simulink model "simulacao1a"  (R2020b)
settings: Solver=VariableStepAuto  StartTime=0.0  StopTime=10  RelTol=1e-3
values from neighbouring files (symbols this model uses):
  b = 0.24    [drone.m]
  B = 0.00029*[1 1 1 1]    [drone.m]
  delta_equilibrium = (Ke(1)*Omega(1) + R(1)*(KQ(1)*Omega(1) + B(1))*Omega(1)/Kt(1))/Vbat    [drone.m]
  J = diag([3.8e-3,3.8e-3,7.1e-3])    [drone.m]
  Jm = 1.4e-5*[1 1 1 1]    [drone.m]
  K = [ Hgain_pd(2) 0             0               0             Hgain_pd(1) 0             0               0 ... (first row only)    [drone.m]
  Ke = 0.0247*[1 1 1 1]    [drone.m]
  KQ = 1.2191e-5*[1 1 1 1]    [drone.m]
  Kt = 0.0247*[1 1 1 1]    [drone.m]
  KT = 3.5897e-5*[1 1 1 1]    [drone.m]
  L = 0.00036*[1 1 1 1]    [drone.m]
  m = 2    [drone.m]
  R = [ cos(target_phi)*cos(target_psi),    cos(target_psi)*sin(target_theta)*sin(target_phi) - sin(target_psi)*cos(target_phi),  cos(target_psi)*sin(target_theta)*cos(target_phi) + sin(target_psi)*sin(target_phi) ... (first row only)    [drone.m]
  Vbat = 15    [drone.m]
libraries: dspmtrx3 x19, vrlib x2
settings Model: Creator=55159  LastModifiedBy=55159
settings DebuggingCC: UnderSpecifiedDimensionMsg=warning

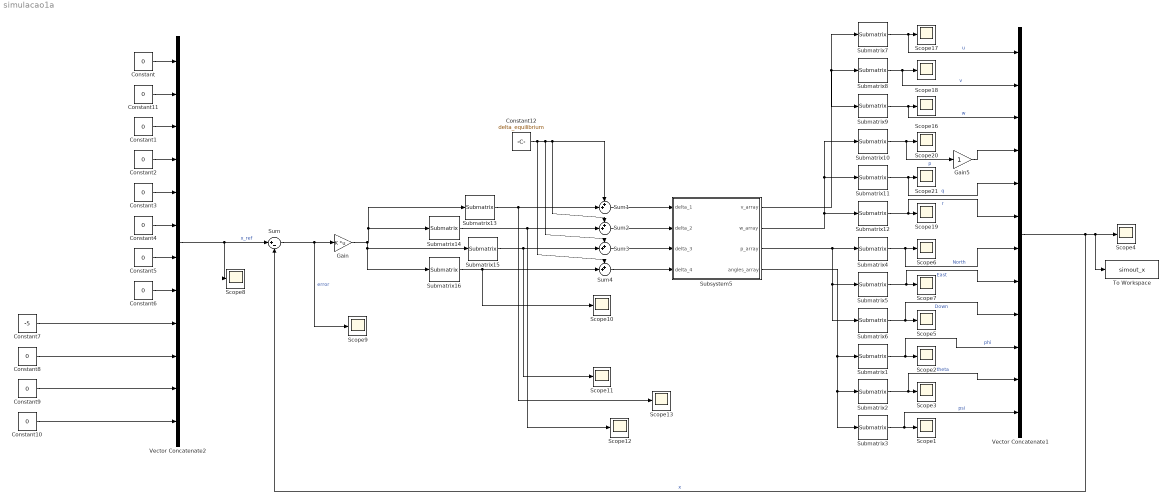
== system simulacao1a ==
  Constant{,1..6,8..11} (11 alike) : Constant  Value=0
  Constant12 : Constant  Value=delta_equilibrium
  Constant7 : Constant  Value=-5
  Gain : Gain  Gain=K  Multiplication=Matrix(K*u) (u vector)
  Gain5 : Gain
  Scope{1..13,16..21} (19 alike) : Scope
  Submatrix{1,4,7,10,13} (5 alike) : dspmtrx3/Submatrix  RowSpan=One row  RowStartMode=Index  RowStartIndex=1  RowEndMode=Last  RowEndIndex=1  ColSpan=One column  ColStartMode=First  ColStartIndex=1  ColEndMode=Last  ColEndIndex=1
  Submatrix11 : dspmtrx3/Submatrix  RowSpan=One row  RowStartMode=Index  RowStartIndex=2  RowEndMode=Last  RowEndIndex=1  ColSpan=One column  ColStartMode=First  ColStartIndex=1  ColEndMode=Last  ColEndIndex=1
  Submatrix12 : dspmtrx3/Submatrix  RowSpan=One row  RowStartMode=Index  RowStartIndex=3  RowEndMode=Last  RowEndIndex=1  ColSpan=One column  ColStartMode=First  ColStartIndex=1  ColEndMode=Last  ColEndIndex=1
  Submatrix14 : dspmtrx3/Submatrix  RowSpan=One row  RowStartMode=Index  RowStartIndex=2  RowEndMode=Last  RowEndIndex=1  ColSpan=One column  ColStartMode=Index  ColStartIndex=1  ColEndMode=Last  ColEndIndex=1
  Submatrix15 : dspmtrx3/Submatrix  RowSpan=One row  RowStartMode=Index  RowStartIndex=3  RowEndMode=Last  RowEndIndex=1  ColSpan=One column  ColStartMode=Index  ColStartIndex=1  ColEndMode=Last  ColEndIndex=1
  Submatrix16 : dspmtrx3/Submatrix  RowSpan=One row  RowStartMode=Index  RowStartIndex=4  RowEndMode=Last  RowEndIndex=1  ColSpan=One column  ColStartMode=Index  ColStartIndex=1  ColEndMode=Last  ColEndIndex=1
  Submatrix2 : dspmtrx3/Submatrix  RowSpan=One row  RowStartMode=Index  RowStartIndex=2  RowEndMode=Last  RowEndIndex=1  ColSpan=One column  ColStartMode=Index  ColStartIndex=1  ColEndMode=Last  ColEndIndex=1
  Submatrix3 : dspmtrx3/Submatrix  RowSpan=One row  RowStartMode=Index  RowStartIndex=3  RowEndMode=Last  RowEndIndex=1  ColSpan=One column  ColStartMode=Index  ColStartIndex=1  ColEndMode=Last  ColEndIndex=1
  Submatrix5 : dspmtrx3/Submatrix  RowSpan=One row  RowStartMode=Index  RowStartIndex=2  RowEndMode=Last  RowEndIndex=1  ColSpan=One column  ColStartMode=First  ColStartIndex=1  ColEndMode=Last  ColEndIndex=1
  Submatrix6 : dspmtrx3/Submatrix  RowSpan=One row  RowStartMode=Index  RowStartIndex=3  RowEndMode=Last  RowEndIndex=1  ColSpan=One column  ColStartMode=First  ColStartIndex=1  ColEndMode=Last  ColEndIndex=1
  Submatrix8 : dspmtrx3/Submatrix  RowSpan=One row  RowStartMode=Index  RowStartIndex=2  RowEndMode=Last  RowEndIndex=1  ColSpan=One column  ColStartMode=First  ColStartIndex=1  ColEndMode=Last  ColEndIndex=1
  Submatrix9 : dspmtrx3/Submatrix  RowSpan=One row  RowStartMode=Index  RowStartIndex=3  RowEndMode=Last  RowEndIndex=1  ColSpan=One column  ColStartMode=First  ColStartIndex=1  ColEndMode=Last  ColEndIndex=1
  Subsystem5 : Subsystem
  Sum : Sum  Inputs=|+-
  Sum{1..4} (4 alike) : Sum  Inputs=++|
  To Workspace : ToWorkspace  VariableName=simout_x  SaveFormat=Timeseries  SampleTime=-1
  Vector Concatenate1 : Concatenate  NumInputs=12
  Vector Concatenate2 : Concatenate  NumInputs=12
  wires:
  Submatrix4/1 -> Vector Concatenate1/7, Scope6/1  "North"
  Submatrix5/1 -> Vector Concatenate1/8, Scope7/1  "East"
  Submatrix6/1 -> Vector Concatenate1/9, Scope5/1  "Down"
  Submatrix8/1 -> Vector Concatenate1/2, Scope18/1  "v"
  Submatrix9/1 -> Vector Concatenate1/3, Scope16/1  "w"
  Submatrix7/1 -> Vector Concatenate1/1, Scope17/1  "u"
  Submatrix12/1 -> Vector Concatenate1/6, Scope19/1  "r"
  Submatrix11/1 -> Vector Concatenate1/5, Scope21/1  "q"
  Submatrix10/1 -> Gain5/1, Scope20/1  "p"
  Subsystem5/4(angles_array) -> Submatrix3/1, Submatrix2/1, Submatrix1/1
  Subsystem5/1(v_array) -> Submatrix7/1, Submatrix9/1, Submatrix8/1
  Subsystem5/3(p_array) -> Submatrix6/1, Submatrix5/1, Submatrix4/1
  Subsystem5/2(w_array) -> Submatrix10/1, Submatrix11/1, Submatrix12/1
  Submatrix2/1 -> Vector Concatenate1/11, Scope3/1  "theta"
  Submatrix3/1 -> Vector Concatenate1/12, Scope1/1  "psi"
  Submatrix1/1 -> Vector Concatenate1/10, Scope2/1  "phi"
  Vector Concatenate1/1 -> Sum/2, To Workspace/1, Scope4/1  "x"
  Vector Concatenate2/1 -> Scope8/1, Sum/1  "x_ref"
  Constant/1 -> Vector Concatenate2/1
  Constant11/1 -> Vector Concatenate2/2
  Constant1/1 -> Vector Concatenate2/3
  Constant2/1 -> Vector Concatenate2/4
  Constant3/1 -> Vector Concatenate2/5
  Constant4/1 -> Vector Concatenate2/6
  Constant5/1 -> Vector Concatenate2/7
  Constant6/1 -> Vector Concatenate2/8
  Constant7/1 -> Vector Concatenate2/9
  Constant8/1 -> Vector Concatenate2/10
  Constant9/1 -> Vector Concatenate2/11
  Constant10/1 -> Vector Concatenate2/12
  Sum/1 -> Scope9/1, Gain/1  "error"
  Gain/1 -> Submatrix16/1, Submatrix15/1, Submatrix13/1, Submatrix14/1
  Sum1/1 -> Subsystem5/1(delta_1)
  Sum4/1 -> Subsystem5/4(delta_4)
  Sum3/1 -> Subsystem5/3(delta_3)
  Sum2/1 -> Subsystem5/2(delta_2)
  Constant12/1 -> Sum1/1, Sum2/1, Sum3/1, Sum4/1
  Submatrix13/1 -> Scope13/1, Sum1/2
  Submatrix14/1 -> Scope12/1, Sum2/2
  Submatrix15/1 -> Scope11/1, Sum3/2
  Submatrix16/1 -> Scope10/1, Sum4/2
  Gain5/1 -> Vector Concatenate1/4

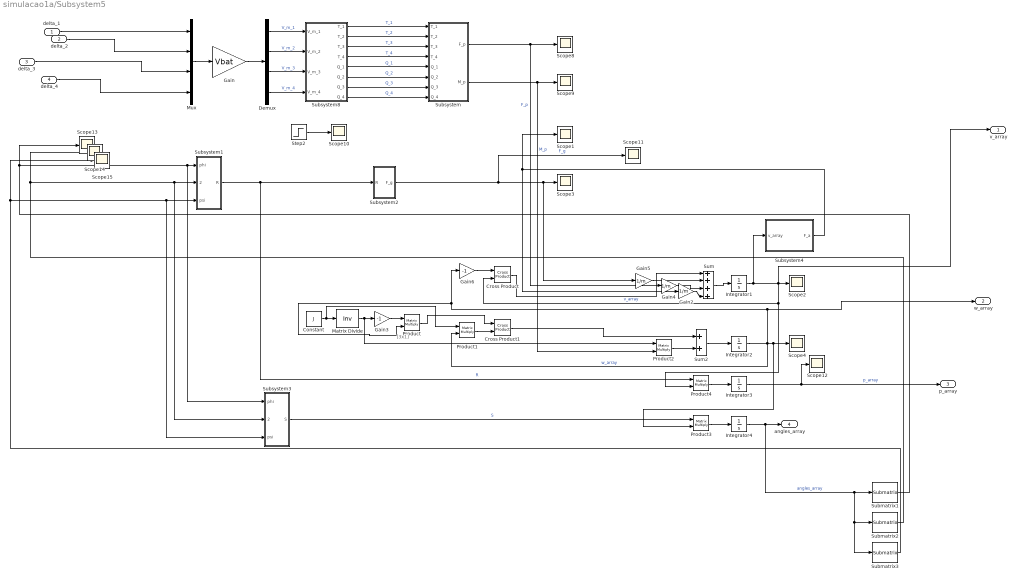
== system simulacao1a/Subsystem5 ==
  note: [3x1]
  delta_1 : Inport
  delta_2 : Inport  Port=2
  delta_3 : Inport  Port=3
  delta_4 : Inport  Port=4
  Constant : Constant  Value=J
  Cross Product : vrlib/Utilities/Cross Product
  Cross Product1 : vrlib/Utilities/Cross Product
  Demux : Demux
  Gain : Gain  Gain=Vbat
  Gain2 : Gain  Gain=1/m
  Gain3 : Gain  Gain=-1
  Gain4 : Gain  Gain=1/m
  Gain5 : Gain  Gain=1/m
  Gain6 : Gain  Gain=-1
  Integrator{1..4} (4 alike) : Integrator
  Matrix Divide : Product  Inputs=/  Multiplication=Matrix(*)
  Mux : Mux
  Product{,1..2,4} (4 alike) : Product  Multiplication=Matrix(*)
  Product3 : Product  Multiplication=Matrix(*)  InputSameDT=on
  Scope{1..4,8..15} (12 alike) : Scope
  Step2 : Step  SampleTime=0
  Submatrix1 : dspmtrx3/Submatrix  RowSpan=One row  RowStartMode=Index  RowStartIndex=1  RowEndMode=Last  RowEndIndex=1  ColSpan=One column  ColStartMode=First  ColStartIndex=1  ColEndMode=Last  ColEndIndex=1
  Submatrix2 : dspmtrx3/Submatrix  RowSpan=One row  RowStartMode=Index  RowStartIndex=2  RowEndMode=Last  RowEndIndex=1  ColSpan=One column  ColStartMode=Index  ColStartIndex=1  ColEndMode=Last  ColEndIndex=1
  Submatrix3 : dspmtrx3/Submatrix  RowSpan=One row  RowStartMode=Index  RowStartIndex=3  RowEndMode=Last  RowEndIndex=1  ColSpan=One column  ColStartMode=Index  ColStartIndex=1  ColEndMode=Last  ColEndIndex=1
  Subsystem : Subsystem
  Subsystem1 : Subsystem
  Subsystem2 : Subsystem
  Subsystem3 : Subsystem
  Subsystem4 : Subsystem
  Subsystem8 : Subsystem
  Sum : Sum  Inputs=++++
  Sum2 : Sum
  v_array : Outport
  w_array : Outport  Port=2
  p_array : Outport  Port=3
  angles_array : Outport  Port=4
  wires:
  Subsystem8/7(Q_3) -> Subsystem/7(Q_3)  "Q_3"
  Sum/1 -> Integrator1/1
  Integrator3/1 -> p_array/1, Scope12/1  "p_array"
  Subsystem/1(F_p) -> Scope8/1, Gain4/1  "F_p"
  Subsystem2/1(F_g) -> Scope11/1, Gain5/1, Scope3/1  "F_g"
  Subsystem4/1(F_a) -> Scope1/1, Gain2/1
  Integrator1/1 -> Subsystem4/1(v_array), v_array/1, Product4/2, Cross Product/2, Scope2/1  "v_array"
  Sum2/1 -> Integrator2/1
  Mux/1 -> Gain/1
  Gain/1 -> Demux/1
  Integrator2/1 -> Product1/2, w_array/1, Product/2, Gain6/1, Product3/2, Scope4/1  "w_array"
  Step2/1 -> Scope10/1
  Demux/3 -> Subsystem8/3(V_m_3)  "V_m_3"
  Subsystem1/1(R) -> Product4/1, Subsystem2/1(R)  "R"
  Gain2/1 -> Sum/4
  Submatrix3/1 -> Scope15/1, Subsystem3/3(psi), Subsystem1/3(psi)
  Subsystem8/1(T_1) -> Subsystem/1(T_1)  "T_1"
  Product4/1 -> Integrator3/1
  Subsystem3/1(S) -> Product3/1  "S"
  Product3/1 -> Integrator4/1
  Demux/1 -> Subsystem8/1(V_m_1)  "V_m_1"
  Demux/4 -> Subsystem8/4(V_m_4)  "V_m_4"
  Subsystem/2(M_p) -> Product2/2, Scope9/1  "M_p"
  Subsystem8/5(Q_1) -> Subsystem/5(Q_1)  "Q_1"
  Matrix Divide/1 -> Product2/1, Gain3/1
  Gain4/1 -> Sum/3
  Gain5/1 -> Sum/2
  Constant/1 -> Product1/1, Matrix Divide/1
  Gain3/1 -> Product/1
  Product1/1 -> Cross Product1/2
  Cross Product/1 -> Sum/1
  delta_3/1 -> Mux/3
  Gain6/1 -> Cross Product/1
  Submatrix2/1 -> Scope14/1, Subsystem3/2(theta), Subsystem1/2(theta)
  Subsystem8/2(T_2) -> Subsystem/2(T_2)  "T_2"
  Subsystem8/3(T_3) -> Subsystem/3(T_3)  "T_3"
  Subsystem8/4(T_4) -> Subsystem/4(T_4)  "T_4"
  Subsystem8/6(Q_2) -> Subsystem/6(Q_2)  "Q_2"
  Product/1 -> Cross Product1/1
  delta_4/1 -> Mux/4
  Subsystem8/8(Q_4) -> Subsystem/8(Q_4)  "Q_4"
  Demux/2 -> Subsystem8/2(V_m_2)  "V_m_2"
  Submatrix1/1 -> Scope13/1, Subsystem3/1(phi), Subsystem1/1(phi)
  Cross Product1/1 -> Sum2/1
  Product2/1 -> Sum2/2
  Integrator4/1 -> Submatrix3/1, Submatrix2/1, Submatrix1/1, angles_array/1  "angles_array"
  delta_1/1 -> Mux/1
  delta_2/1 -> Mux/2

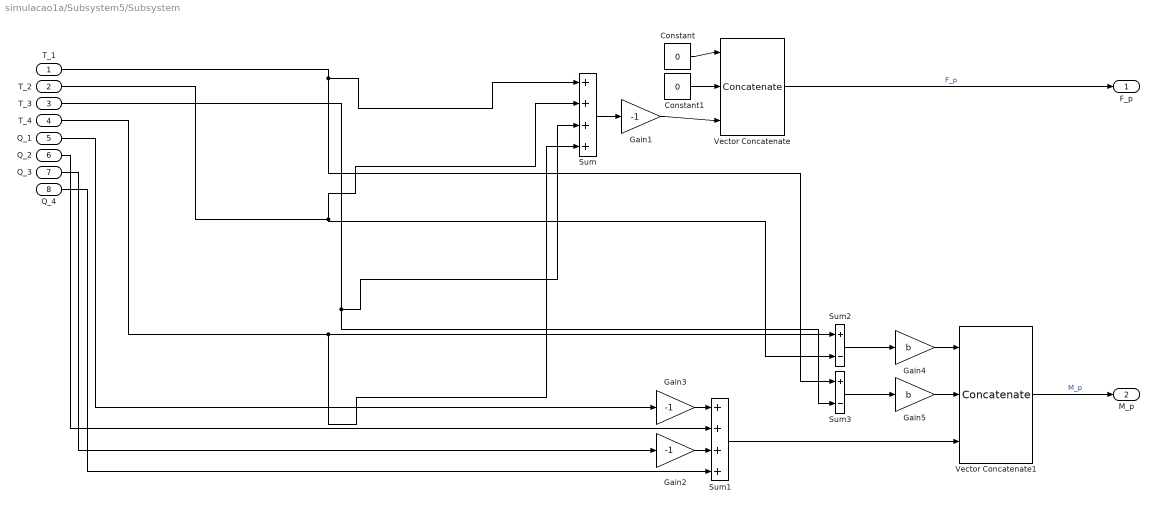
== system simulacao1a/Subsystem5/Subsystem ==
  T_1 : Inport
  T_2 : Inport  Port=2
  T_3 : Inport  Port=3
  T_4 : Inport  Port=4
  Q_1 : Inport  Port=5
  Q_2 : Inport  Port=6
  Q_3 : Inport  Port=7
  Q_4 : Inport  Port=8
  Constant : Constant  Value=0
  Constant1 : Constant  Value=0
  Gain1 : Gain  Gain=-1
  Gain2 : Gain  Gain=-1
  Gain3 : Gain  Gain=-1
  Gain4 : Gain  Gain=b
  Gain5 : Gain  Gain=b
  Sum : Sum  Inputs=++++
  Sum1 : Sum  Inputs=++++
  Sum2 : Sum  Inputs=+-
  Sum3 : Sum  Inputs=+-
  Vector Concatenate : Concatenate  NumInputs=3
  Vector Concatenate1 : Concatenate  NumInputs=3
  F_p : Outport  PortDimensions=[3 1]
  M_p : Outport  Port=2  PortDimensions=[3 1]
  wires:
  T_4/1 -> Sum/4, Sum2/1
  Q_1/1 -> Gain3/1
  Gain4/1 -> Vector Concatenate1/1
  T_3/1 -> Sum3/2, Sum/3
  T_1/1 -> Sum3/1, Sum/1
  Gain2/1 -> Sum1/3
  Constant1/1 -> Vector Concatenate/2
  Gain3/1 -> Sum1/1
  Sum2/1 -> Gain4/1
  Sum/1 -> Gain1/1
  Gain5/1 -> Vector Concatenate1/2
  Gain1/1 -> Vector Concatenate/3
  Constant/1 -> Vector Concatenate/1
  Vector Concatenate/1 -> F_p/1  "F_p"
  T_2/1 -> Sum/2, Sum2/2
  Sum1/1 -> Vector Concatenate1/3
  Sum3/1 -> Gain5/1
  Vector Concatenate1/1 -> M_p/1  "M_p"
  Q_2/1 -> Sum1/2
  Q_3/1 -> Gain2/1
  Q_4/1 -> Sum1/4

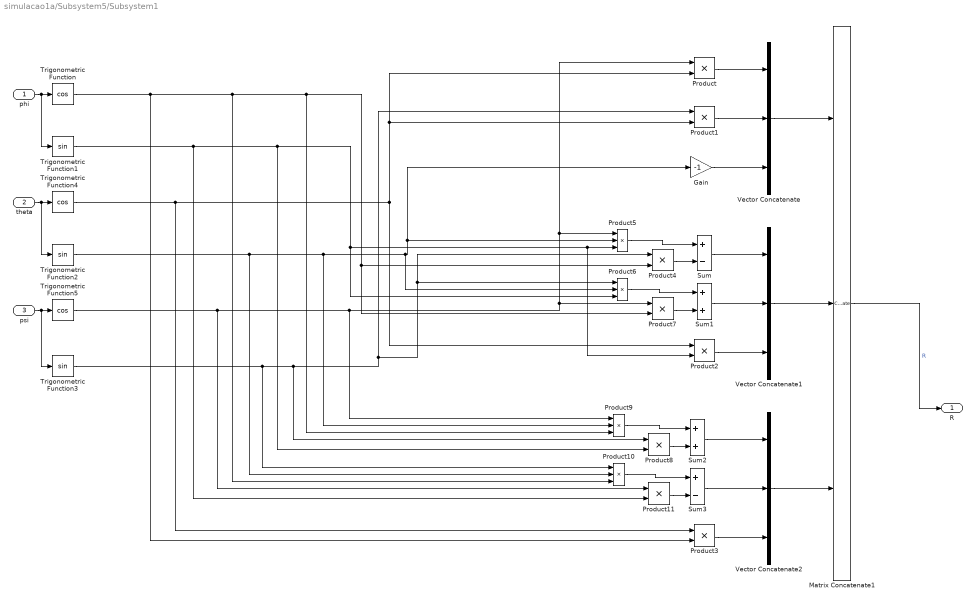
== system simulacao1a/Subsystem5/Subsystem1 ==
  phi : Inport
  theta : Inport  Port=2
  psi : Inport  Port=3
  Gain : Gain  Gain=-1
  Matrix Concatenate1 : Concatenate  NumInputs=3  Mode=Multidimensional array  ConcatenateDimension=2
  Product{,1..4,7..8,11} (8 alike) : Product
  Product{5..6,9..10} (4 alike) : Product  Inputs=3
  Sum : Sum  Inputs=+-
  Sum1 : Sum
  Sum2 : Sum
  Sum3 : Sum  Inputs=+-
  Trigonometric Function : Trigonometry  Operator=cos
  Trigonometric Function1 : Trigonometry
  Trigonometric Function2 : Trigonometry
  Trigonometric Function3 : Trigonometry
  Trigonometric Function4 : Trigonometry  Operator=cos
  Trigonometric Function5 : Trigonometry  Operator=cos
  Vector Concatenate : Concatenate  NumInputs=3  Mode=Multidimensional array
  Vector Concatenate1 : Concatenate  NumInputs=3  Mode=Multidimensional array
  Vector Concatenate2 : Concatenate  NumInputs=3  Mode=Multidimensional array
  R : Outport  PortDimensions=[3 3]
  wires:
  phi/1 -> Trigonometric Function1/1, Trigonometric Function/1
  theta/1 -> Trigonometric Function4/1, Trigonometric Function2/1
  psi/1 -> Trigonometric Function3/1, Trigonometric Function5/1
  Product/1 -> Vector Concatenate/1
  Product1/1 -> Vector Concatenate/2
  Sum1/1 -> Vector Concatenate1/2
  Sum/1 -> Vector Concatenate1/1
  Sum2/1 -> Vector Concatenate2/1
  Gain/1 -> Vector Concatenate/3
  Trigonometric Function5/1 -> Product11/1, Product9/1, Product7/1, Product5/1, Product/1
  Trigonometric Function4/1 -> Product3/1, Product1/2, Product/2, Product2/1
  Trigonometric Function3/1 -> Product10/1, Product8/1, Product6/1, Product4/1, Product1/1
  Product4/1 -> Sum/2
  Product5/1 -> Sum/1
  Trigonometric Function2/1 -> Product10/2, Product9/2, Product6/2, Gain/1, Product5/2
  Trigonometric Function1/1 -> Product11/2, Product8/2, Product6/3, Product5/3, Product2/2
  Trigonometric Function/1 -> Product3/2, Product10/3, Product9/3, Product7/2, Product4/2
  Product6/1 -> Sum1/1
  Product7/1 -> Sum1/2
  Product2/1 -> Vector Concatenate1/3
  Product9/1 -> Sum2/1
  Product10/1 -> Sum3/1
  Product8/1 -> Sum2/2
  Product11/1 -> Sum3/2
  Product3/1 -> Vector Concatenate2/3
  Vector Concatenate/1 -> Matrix Concatenate1/1
  Vector Concatenate1/1 -> Matrix Concatenate1/2
  Vector Concatenate2/1 -> Matrix Concatenate1/3
  Matrix Concatenate1/1 -> R/1  "R"
  Sum3/1 -> Vector Concatenate2/2

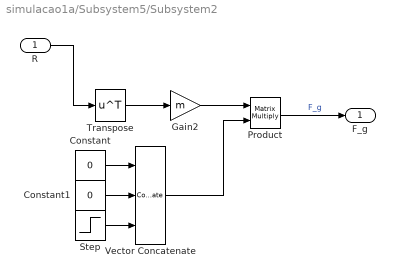
== system simulacao1a/Subsystem5/Subsystem2 ==
  R : Inport
  Constant : Constant  Value=0
  Constant1 : Constant  Value=0
  Gain2 : Gain  Gain=m
  Product : Product  Multiplication=Matrix(*)
  Step : Step  Time=0  After=9.81  SampleTime=0
  Transpose : Math  Operator=transpose  SaturateOnIntegerOverflow=on
  Vector Concatenate : Concatenate  NumInputs=3
  F_g : Outport
  wires:
  Constant/1 -> Vector Concatenate/1
  R/1 -> Transpose/1
  Gain2/1 -> Product/1
  Constant1/1 -> Vector Concatenate/2
  Vector Concatenate/1 -> Product/2
  Product/1 -> F_g/1  "F_g"
  Transpose/1 -> Gain2/1
  Step/1 -> Vector Concatenate/3

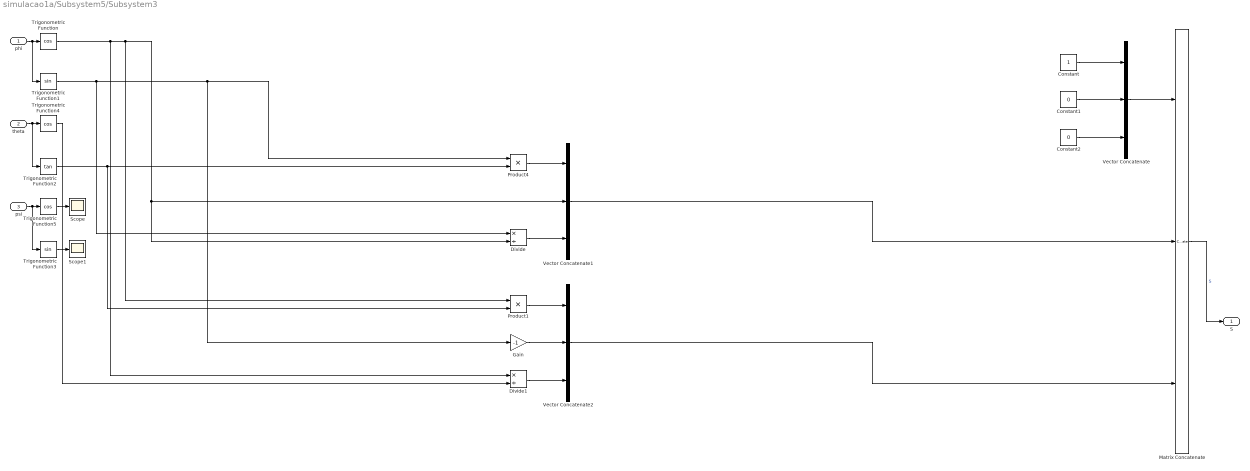
== system simulacao1a/Subsystem5/Subsystem3 ==
  phi : Inport
  theta : Inport  Port=2
  psi : Inport  Port=3
  Constant : Constant
  Constant1 : Constant  Value=0
  Constant2 : Constant  Value=0
  Divide : Product  Inputs=*/
  Divide1 : Product  Inputs=*/
  Gain : Gain  Gain=-1
  Matrix Concatenate : Concatenate  NumInputs=3  Mode=Multidimensional array  ConcatenateDimension=2
  Product1 : Product
  Product4 : Product
  Scope : Scope
  Scope1 : Scope
  Trigonometric Function : Trigonometry  Operator=cos
  Trigonometric Function1 : Trigonometry
  Trigonometric Function2 : Trigonometry  Operator=tan
  Trigonometric Function3 : Trigonometry
  Trigonometric Function4 : Trigonometry  Operator=cos
  Trigonometric Function5 : Trigonometry  Operator=cos
  Vector Concatenate : Concatenate  NumInputs=3
  Vector Concatenate1 : Concatenate  NumInputs=3
  Vector Concatenate2 : Concatenate  NumInputs=3
  S : Outport  PortDimensions=[3 3]
  wires:
  Matrix Concatenate/1 -> S/1  "S"
  phi/1 -> Trigonometric Function1/1, Trigonometric Function/1
  theta/1 -> Trigonometric Function4/1, Trigonometric Function2/1
  psi/1 -> Trigonometric Function3/1, Trigonometric Function5/1
  Divide/1 -> Vector Concatenate1/3
  Constant/1 -> Vector Concatenate/1
  Constant1/1 -> Vector Concatenate/2
  Constant2/1 -> Vector Concatenate/3
  Trigonometric Function/1 -> Divide1/1, Product1/1, Divide/2, Vector Concatenate1/2
  Product4/1 -> Vector Concatenate1/1
  Divide1/1 -> Vector Concatenate2/3
  Gain/1 -> Vector Concatenate2/2
  Product1/1 -> Vector Concatenate2/1
  Trigonometric Function1/1 -> Divide/1, Gain/1, Product4/1
  Trigonometric Function2/1 -> Product1/2, Product4/2
  Trigonometric Function4/1 -> Divide1/2
  Trigonometric Function5/1 -> Scope/1
  Trigonometric Function3/1 -> Scope1/1
  Vector Concatenate/1 -> Matrix Concatenate/1
  Vector Concatenate1/1 -> Matrix Concatenate/2
  Vector Concatenate2/1 -> Matrix Concatenate/3

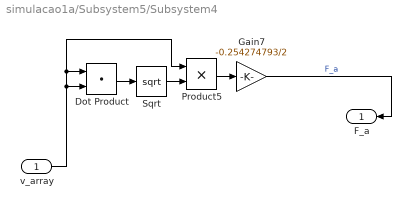
== system simulacao1a/Subsystem5/Subsystem4 ==
  v_array : Inport
  Dot Product : DotProduct  InputSameDT=on  OutDataTypeStr=Inherit: Inherit via internal rule
  Gain7 : Gain  Gain=-0.254274793/2
  Product5 : Product
  Sqrt : Sqrt  SaturateOnIntegerOverflow=on
  F_a : Outport  PortDimensions=[3 1]
  wires:
  v_array/1 -> Dot Product/2, Product5/1, Dot Product/1
  Product5/1 -> Gain7/1
  Sqrt/1 -> Product5/2
  Dot Product/1 -> Sqrt/1
  Gain7/1 -> F_a/1  "F_a"

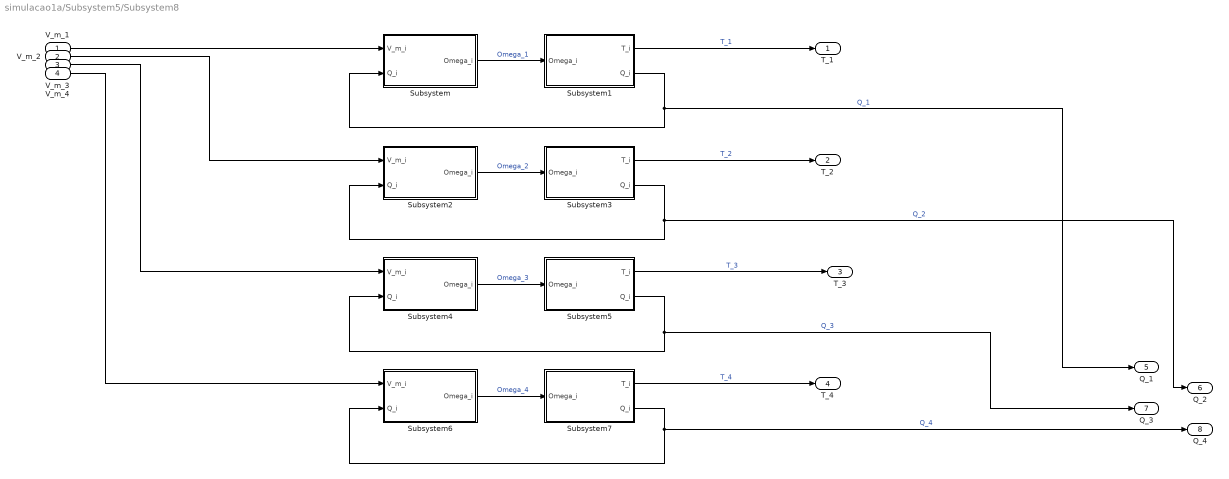
== system simulacao1a/Subsystem5/Subsystem8 ==
  V_m_1 : Inport
  V_m_2 : Inport  Port=2
  V_m_3 : Inport  Port=3
  V_m_4 : Inport  Port=4
  Subsystem : Subsystem
  Subsystem1 : Subsystem
  Subsystem2 : Subsystem
  Subsystem3 : Subsystem
  Subsystem4 : Subsystem
  Subsystem5 : Subsystem
  Subsystem6 : Subsystem
  Subsystem7 : Subsystem
  T_1 : Outport
  T_2 : Outport  Port=2
  T_3 : Outport  Port=3
  T_4 : Outport  Port=4
  Q_1 : Outport  Port=5
  Q_2 : Outport  Port=6
  Q_3 : Outport  Port=7
  Q_4 : Outport  Port=8
  wires:
  Subsystem6/1(Omega_i) -> Subsystem7/1(Omega_i)  "Omega_4"
  Subsystem3/2(Q_i) -> Q_2/1, Subsystem2/2(Q_i)  "Q_2"
  Subsystem7/2(Q_i) -> Subsystem6/2(Q_i), Q_4/1  "Q_4"
  Subsystem1/2(Q_i) -> Q_1/1, Subsystem/2(Q_i)  "Q_1"
  Subsystem/1(Omega_i) -> Subsystem1/1(Omega_i)  "Omega_1"
  V_m_1/1 -> Subsystem/1(V_m_i)
  V_m_2/1 -> Subsystem2/1(V_m_i)
  Subsystem1/1(T_i) -> T_1/1  "T_1"
  Subsystem5/2(Q_i) -> Q_3/1, Subsystem4/2(Q_i)  "Q_3"
  Subsystem4/1(Omega_i) -> Subsystem5/1(Omega_i)  "Omega_3"
  Subsystem2/1(Omega_i) -> Subsystem3/1(Omega_i)  "Omega_2"
  Subsystem7/1(T_i) -> T_4/1  "T_4"
  Subsystem5/1(T_i) -> T_3/1  "T_3"
  V_m_3/1 -> Subsystem4/1(V_m_i)
  Subsystem3/1(T_i) -> T_2/1  "T_2"
  V_m_4/1 -> Subsystem6/1(V_m_i)

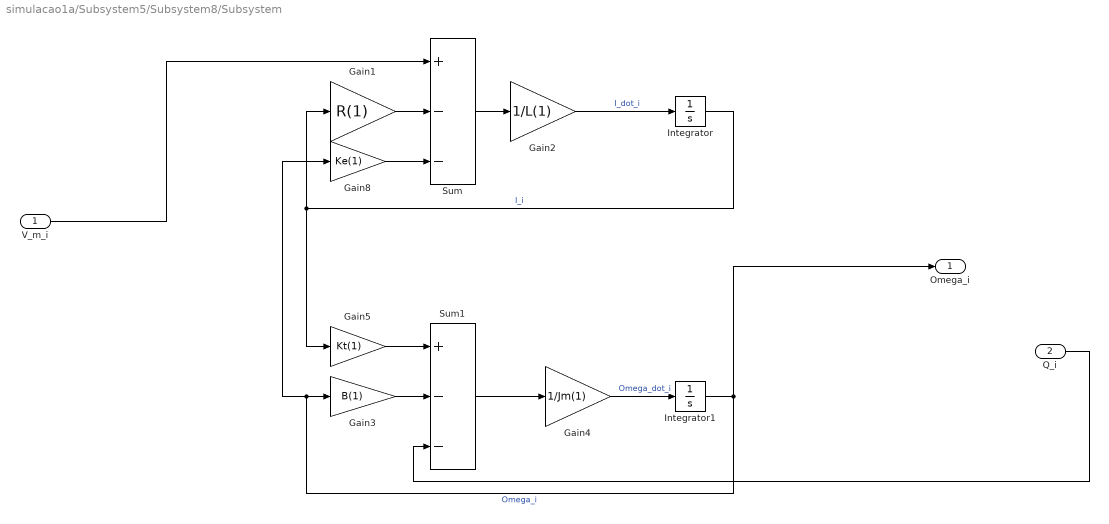
== system simulacao1a/Subsystem5/Subsystem8/Subsystem ==
  V_m_i : Inport
  Q_i : Inport  Port=2
  Gain1 : Gain  Gain=R(1)
  Gain2 : Gain  Gain=1/L(1)
  Gain3 : Gain  Gain=B(1)
  Gain4 : Gain  Gain=1/Jm(1)
  Gain5 : Gain  Gain=Kt(1)
  Gain8 : Gain  Gain=Ke(1)
  Integrator : Integrator
  Integrator1 : Integrator
  Sum : Sum  Inputs=+--
  Sum1 : Sum  Inputs=+--
  Omega_i : Outport
  wires:
  Gain4/1 -> Integrator1/1  "Omega_dot_i"
  V_m_i/1 -> Sum/1
  Integrator1/1 -> Omega_i/1, Gain8/1, Gain3/1  "Omega_i"
  Sum/1 -> Gain2/1
  Q_i/1 -> Sum1/3
  Sum1/1 -> Gain4/1
  Gain1/1 -> Sum/2
  Gain8/1 -> Sum/3
  Integrator/1 -> Gain1/1, Gain5/1  "I_i"
  Gain5/1 -> Sum1/1
  Gain3/1 -> Sum1/2
  Gain2/1 -> Integrator/1  "I_dot_i"

== system simulacao1a/Subsystem5/Subsystem8/Subsystem1 ==
  Omega_i : Inport
  Gain6 : Gain  Gain=KT(1)
  Gain7 : Gain  Gain=KQ(1)
  Math Function : Math  Operator=square  SaturateOnIntegerOverflow=on
  T_i : Outport
  Q_i : Outport  Port=2
  wires:
  Gain6/1 -> T_i/1  "T_i"
  Math Function/1 -> Gain7/1, Gain6/1
  Omega_i/1 -> Math Function/1
  Gain7/1 -> Q_i/1  "Q_i"

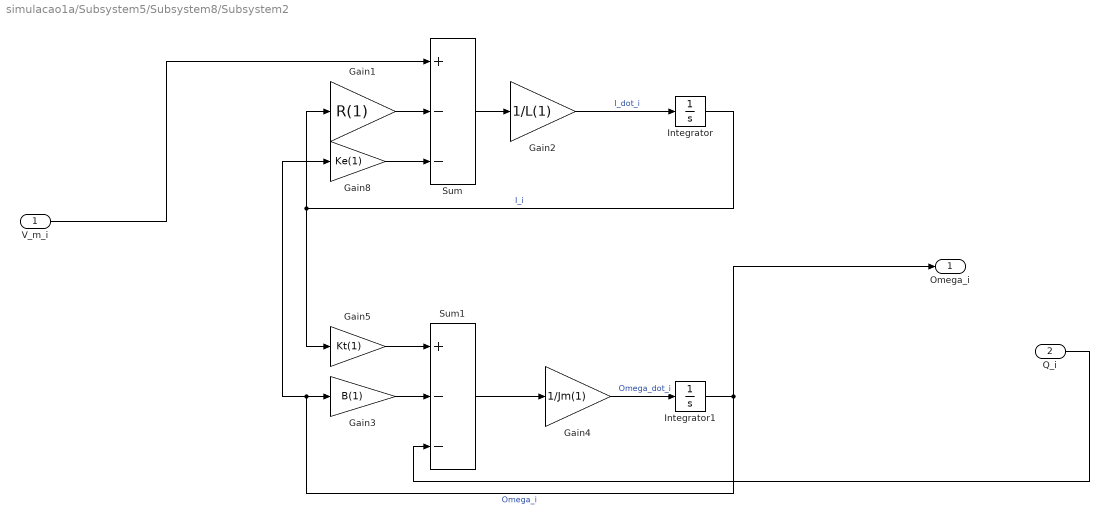
== system simulacao1a/Subsystem5/Subsystem8/Subsystem2 ==
  V_m_i : Inport
  Q_i : Inport  Port=2
  Gain1 : Gain  Gain=R(1)
  Gain2 : Gain  Gain=1/L(1)
  Gain3 : Gain  Gain=B(1)
  Gain4 : Gain  Gain=1/Jm(1)
  Gain5 : Gain  Gain=Kt(1)
  Gain8 : Gain  Gain=Ke(1)
  Integrator : Integrator
  Integrator1 : Integrator
  Sum : Sum  Inputs=+--
  Sum1 : Sum  Inputs=+--
  Omega_i : Outport
  wires:
  Gain4/1 -> Integrator1/1  "Omega_dot_i"
  V_m_i/1 -> Sum/1
  Integrator1/1 -> Omega_i/1, Gain8/1, Gain3/1  "Omega_i"
  Sum/1 -> Gain2/1
  Q_i/1 -> Sum1/3
  Sum1/1 -> Gain4/1
  Gain1/1 -> Sum/2
  Gain8/1 -> Sum/3
  Integrator/1 -> Gain1/1, Gain5/1  "I_i"
  Gain5/1 -> Sum1/1
  Gain3/1 -> Sum1/2
  Gain2/1 -> Integrator/1  "I_dot_i"

== system simulacao1a/Subsystem5/Subsystem8/Subsystem3 ==
  Omega_i : Inport
  Gain6 : Gain  Gain=KT(1)
  Gain7 : Gain  Gain=KQ(1)
  Math Function : Math  Operator=square  SaturateOnIntegerOverflow=on
  T_i : Outport
  Q_i : Outport  Port=2
  wires:
  Gain6/1 -> T_i/1  "T_i"
  Math Function/1 -> Gain7/1, Gain6/1
  Omega_i/1 -> Math Function/1
  Gain7/1 -> Q_i/1  "Q_i"

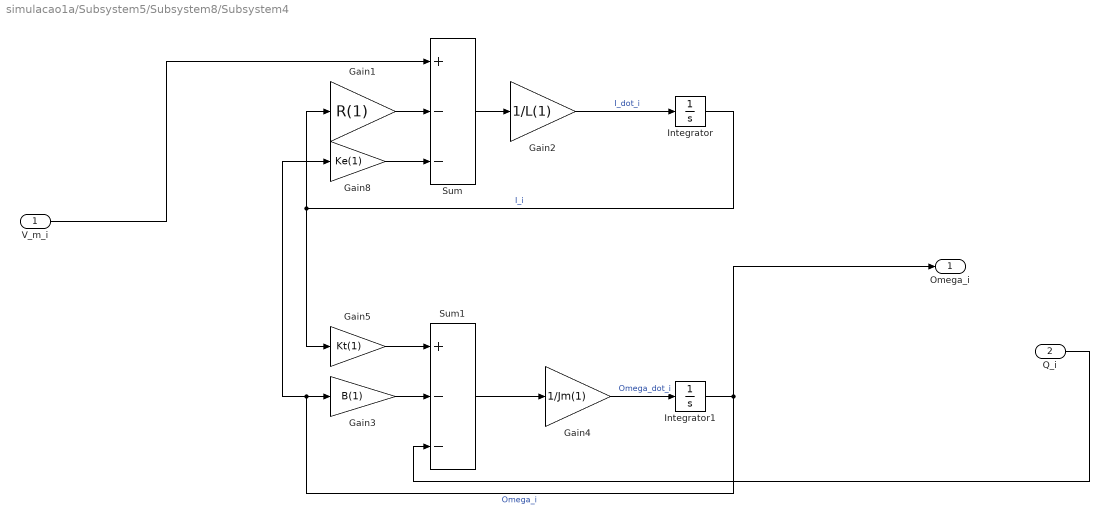
== system simulacao1a/Subsystem5/Subsystem8/Subsystem4 ==
  V_m_i : Inport
  Q_i : Inport  Port=2
  Gain1 : Gain  Gain=R(1)
  Gain2 : Gain  Gain=1/L(1)
  Gain3 : Gain  Gain=B(1)
  Gain4 : Gain  Gain=1/Jm(1)
  Gain5 : Gain  Gain=Kt(1)
  Gain8 : Gain  Gain=Ke(1)
  Integrator : Integrator
  Integrator1 : Integrator
  Sum : Sum  Inputs=+--
  Sum1 : Sum  Inputs=+--
  Omega_i : Outport
  wires:
  Gain4/1 -> Integrator1/1  "Omega_dot_i"
  V_m_i/1 -> Sum/1
  Integrator1/1 -> Omega_i/1, Gain8/1, Gain3/1  "Omega_i"
  Sum/1 -> Gain2/1
  Q_i/1 -> Sum1/3
  Sum1/1 -> Gain4/1
  Gain1/1 -> Sum/2
  Gain8/1 -> Sum/3
  Integrator/1 -> Gain1/1, Gain5/1  "I_i"
  Gain5/1 -> Sum1/1
  Gain3/1 -> Sum1/2
  Gain2/1 -> Integrator/1  "I_dot_i"

== system simulacao1a/Subsystem5/Subsystem8/Subsystem5 ==
  Omega_i : Inport
  Gain6 : Gain  Gain=KT(1)
  Gain7 : Gain  Gain=KQ(1)
  Math Function : Math  Operator=square  SaturateOnIntegerOverflow=on
  T_i : Outport
  Q_i : Outport  Port=2
  wires:
  Gain6/1 -> T_i/1  "T_i"
  Math Function/1 -> Gain7/1, Gain6/1
  Omega_i/1 -> Math Function/1
  Gain7/1 -> Q_i/1  "Q_i"

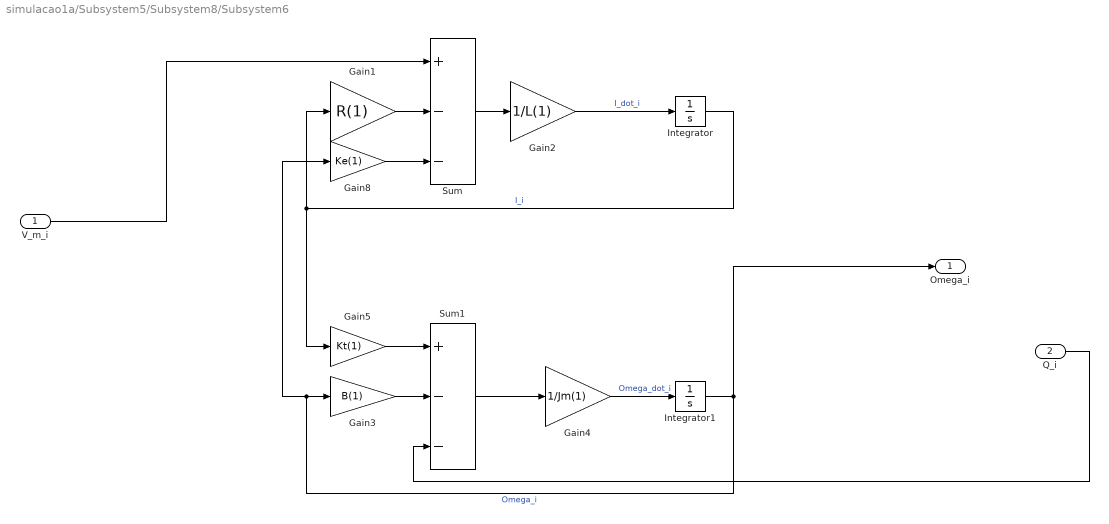
== system simulacao1a/Subsystem5/Subsystem8/Subsystem6 ==
  V_m_i : Inport
  Q_i : Inport  Port=2
  Gain1 : Gain  Gain=R(1)
  Gain2 : Gain  Gain=1/L(1)
  Gain3 : Gain  Gain=B(1)
  Gain4 : Gain  Gain=1/Jm(1)
  Gain5 : Gain  Gain=Kt(1)
  Gain8 : Gain  Gain=Ke(1)
  Integrator : Integrator
  Integrator1 : Integrator
  Sum : Sum  Inputs=+--
  Sum1 : Sum  Inputs=+--
  Omega_i : Outport
  wires:
  Gain4/1 -> Integrator1/1  "Omega_dot_i"
  V_m_i/1 -> Sum/1
  Integrator1/1 -> Omega_i/1, Gain8/1, Gain3/1  "Omega_i"
  Sum/1 -> Gain2/1
  Q_i/1 -> Sum1/3
  Sum1/1 -> Gain4/1
  Gain1/1 -> Sum/2
  Gain8/1 -> Sum/3
  Integrator/1 -> Gain1/1, Gain5/1  "I_i"
  Gain5/1 -> Sum1/1
  Gain3/1 -> Sum1/2
  Gain2/1 -> Integrator/1  "I_dot_i"

== system simulacao1a/Subsystem5/Subsystem8/Subsystem7 ==
  Omega_i : Inport
  Gain6 : Gain  Gain=KT(1)
  Gain7 : Gain  Gain=KQ(1)
  Math Function : Math  Operator=square  SaturateOnIntegerOverflow=on
  T_i : Outport
  Q_i : Outport  Port=2
  wires:
  Gain6/1 -> T_i/1  "T_i"
  Math Function/1 -> Gain7/1, Gain6/1
  Omega_i/1 -> Math Function/1
  Gain7/1 -> Q_i/1  "Q_i"
